simulink model "fullwave_rectifier_usingSCR"  (Simulink 8.3)
settings: Solver=ode23tb  StartTime=0.0  StopTime=2  RelTol=1e-3
libraries: powerlib x10
settings Model: Creator=NILIMESH GHOSH  LastModifiedBy=NILIMESH GHOSH
settings DataIOCC: SignalLoggingSaveFormat=Dataset
settings DebuggingCC: UnderspecifiedInitializationDetection=Simplified  StateNameClashWarn=none
settings GRTTargetCC: CombineOutputUpdateFcns=on  GRTInterface=off

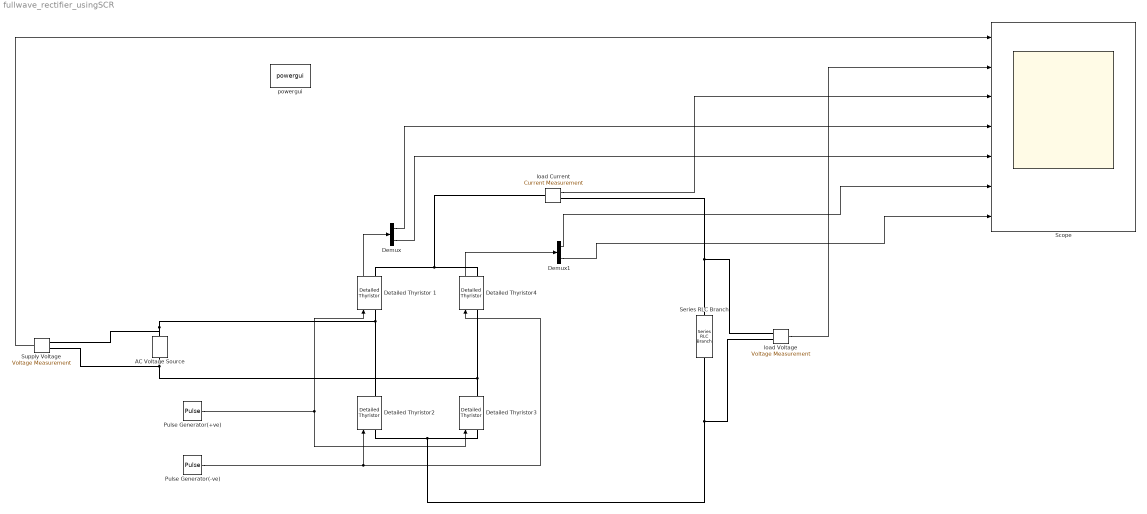
== system fullwave_rectifier_usingSCR ==
  AC Voltage Source : powerlib/Electrical Sources/AC Voltage Source  Amplitude=100  Phase=0  Frequency=50  SampleTime=0  Measurements=None
  Demux : Demux  Outputs=2
  Demux1 : Demux  Outputs=2
  Detailed Thyristor 1 : powerlib/Power Electronics/Detailed Thyristor  Ron=0.001  Lon=1e-3  Vf=0.8  IL=0.1  Tq=100e-6  IC=0  Rs=500  Cs=250e-9  Measurements=on
  Detailed Thyristor2 : powerlib/Power Electronics/Detailed Thyristor  Ron=0.001  Lon=1e-3  Vf=0.8  IL=0.1  Tq=100e-6  IC=0  Rs=500  Cs=250e-9  Measurements=on
  Detailed Thyristor3 : powerlib/Power Electronics/Detailed Thyristor  Ron=0.001  Lon=1e-3  Vf=0.8  IL=0.1  Tq=100e-6  IC=0  Rs=500  Cs=250e-9  Measurements=on
  Detailed Thyristor4 : powerlib/Power Electronics/Detailed Thyristor  Ron=0.001  Lon=1e-3  Vf=0.8  IL=0.1  Tq=100e-6  IC=0  Rs=500  Cs=250e-9  Measurements=on
  Pulse Generator(+ve) : DiscretePulseGenerator  PulseType=Time based  Period=20e-3  PulseWidth=5  PhaseDelay=3e-3  SampleTime=0  VectorParams1D=off
  Pulse Generator(-ve) : DiscretePulseGenerator  PulseType=Time based  Period=20e-3  PulseWidth=5  PhaseDelay=13e-3  VectorParams1D=off
  Scope : Scope  NumInputPorts=7
      settings: TickLabels=on  YMin=-150~-1.11838e-15~-8.40148e-17~-1~-1.36391e-13~-1~-1.36391e-13  YMax=200~-1.01186e-15~-7.60134e-17~1~-1.23401e-13~1~-1.23401e-13
  Series RLC Branch : powerlib/Elements/Series RLC Branch  LConnTagsString=__new0  RConnTagsString=__new0  BranchType=R  Resistance=1  Inductance=1e-3  SetiL0=off  InitialCurrent=0  Capacitance=1e-6  Setx0=off  InitialVoltage=0  Measurements=None
  Supply Voltage : powerlib/Measurements/Voltage Measurement  PhasorSimulation=off  OutputType=Complex  PSBequivalent=0
  "load Current " : powerlib/Measurements/Current Measurement  PhasorSimulation=off  OutputType=Complex  PSBequivalent=0
  "load Voltage " : powerlib/Measurements/Voltage Measurement  PhasorSimulation=off  OutputType=Complex  PSBequivalent=0
  powergui : powerlib/powergui  Priority=1  SimulationMode=Continuous  SolverType=Tustin  SampleTime=50e-6  frequency=60  SPID=off  DisableSnubberDevices=off  DisableRonSwitches=off  DisableVfSwitches=off  SwTol=0  Interpol=off  DisplayEquations=off  Ts=0  methode=off  frequencyindice=50  Pbase=100e6  ErrMax=1e-4  Iterations=50  UnitsV=kV  UnitsW=MW  FunctionMessages=off  echomessages=off  HookPort=off  EnableUseOfTLC=off  x0status=blocks  RestoreLinks=warning  ResistiveCurrentMeasurement=off  Frange=[0:2:500]  Ylog=off  Xlog=on  ShowGrid=off  save=off  variable=ZData  structure=0  ZoomFFT=off  StartTime=0.0  cycles=1  DisplayStyle=1  fundamental=60  FreqAxis=off  MaxFrequency=1000  frequencyindicesteady=1  RmsSteady=1  display=off
  wires:
  Pulse Generator(+ve)/1 -> Detailed Thyristor3/1, Detailed Thyristor 1/1
  Pulse Generator(-ve)/1 -> Detailed Thyristor2/1, Detailed Thyristor4/1
  Supply Voltage/1 -> Scope/1
  "load Voltage "/1 -> Scope/2
  "load Current "/1 -> Scope/3
  Detailed Thyristor 1/1 -> Demux/1
  Demux/1 -> Scope/4
  Demux/2 -> Scope/5
  Detailed Thyristor4/1 -> Demux1/1
  Demux1/1 -> Scope/6
  Demux1/2 -> Scope/7
  connections:
  Series RLC Branch/LConn1 -- "load Current "/RConn1 -- "load Voltage "/LConn1
  Detailed Thyristor2/LConn1 -- Series RLC Branch/RConn1 -- "load Voltage "/LConn2 -- Detailed Thyristor3/LConn1
  Detailed Thyristor2/RConn1 -- Supply Voltage/LConn1 -- AC Voltage Source/RConn1 -- Detailed Thyristor 1/LConn1
  Detailed Thyristor3/RConn1 -- Detailed Thyristor4/LConn1 -- Supply Voltage/LConn2 -- AC Voltage Source/LConn1
  Detailed Thyristor 1/RConn1 -- Detailed Thyristor4/RConn1 -- "load Current "/LConn1
